simulink model "master_thesis_simulink"  (R2022a)
settings: Solver=VariableStepAuto  StartTime=0.0  StopTime=p_0p.time(end)  FixedStep=0.001  RelTol=1e-3
values from neighbouring files (symbols this model uses):
  markers_forearm = [0.00210510253906 -0.143263397217 -0.00798474121094]    [markers_forearm.mat]
  markers_shoulder = [0.010127746582 -0.151647644043 -0.0119686279297]    [markers_shoulder.mat]
undefined symbols (not defined in the file or in its folder): arm, DiscIntNeverNeededParam, Discrete, ekf, kf, LS, m, markers_hand, n, noise, q0, q0_LS, q0_model, sample_Time, selected, state_observer, Time, tSh_0_0Conf, X, Y, Z
libraries: sm_lib x2029, nesl_utility x1553, robotlib x75, ctrlSharedLib x8
(part 7 of 70)

== system master_thesis_simulink/Experiments/S2_F0_H2/Experiments/KF ==
  p_0' : Inport
  v_0' : Inport  Port=2
  Action Port : ActionPort
  Discrete State-Space : DiscreteStateSpace  Commented=on  A=kf.F  B=kf.G  C=kf.H  D=kf.J  InitialCondition=q0_model - kf.q_eq  SampleTime=sample_Time
  Kalman Filter : MATLAB Function  Commented=on  TreatAsAtomicUnit=on
  Kalman Filter1 : ctrlSharedLib/Kalman Filter  TimeDomain=Discrete-Time  UseCurrentEstimator=on  ModelSource=Individual A, B, C, D matrices  ModelSourceVariable=ss(0.95,1,1,0,1)  A=kf.F  B=kf.G  C=kf.H  D=kf.J  NumberOfStates=1  NumberOfInputs=1  NumberOfOutputs=1  InitialEstimateSource=Dialog  X0=kf.Delta_q0  P0=kf.P0  UseK=off  UseGH=off  NumberOfProcessNoiseInputs=1  G=1  TimeInvariantG=on  H=0  TimeInvariantH=on  Q=noise.Q  TimeInvariantQ=on  R=noise.R  TimeInvariantR=on  N=0  TimeInvariantN=on  AddInputPort=on  AddEnablePort=off  OutputEstimatedY=off  OutputP=off  Ts=sample_Time
  MATLAB Function : MATLAB Function  Commented=on  TreatAsAtomicUnit=on
  R : RandomNumber  Commented=on  Variance=diag(noise.R)  Seed=noise.R_seed  SampleTime=sample_Time
  Scope : Scope  NumInputPorts=2
  Sum1 : Sum  Commented=on  Inputs=++|
  Sum2 : Sum  Commented=on  Inputs=++|
  Sum3 : Sum  Inputs=|+-
  Sum4 : Sum  Inputs=++|
  Sum5 : Sum  Commented=on  Inputs=|++
  Sum6 : Sum  Inputs=|+-
  Terminator1 : Terminator  Commented=on
  Terminator2 : Terminator
  Terminator3 : Terminator
  To Workspace1 : ToWorkspace  VariableName=qk_kf  SaveFormat=Structure With Time  SampleTime=-1
  p_eq : Constant  Value=kf.p_eq  SampleTime=sample_Time
  q_eq : Constant  Commented=on  Value=kf.q_eq  SampleTime=sample_Time
  q_eq1 : Constant  Value=kf.q_eq  SampleTime=sample_Time
  trial : Subsystem  Commented=on
  u_eq : Constant  Value=kf.u_eq  SampleTime=sample_Time
  q_KF : Outport
  wires:
  v_0'/1 -> Sum3/1
  u_eq/1 -> Sum3/2  "u_eqk"
  Sum3/1 -> Kalman Filter1/1, Kalman Filter/2(Delta_uk), trial/1(Delta uk), Sum5/2  "Delta _uk"
  Discrete State-Space/1 -> Sum1/2
  R/1 -> Sum1/1
  Kalman Filter/1(Delta_qk) -> Sum2/2  "Delta qk"
  q_eq/1 -> Sum2/1
  Kalman Filter/2(Pk) -> Terminator1/1
  Sum2/1 -> Scope/1  "kf"
  trial/1(q_OBS) -> Terminator2/1
  trial/2(q_KF) -> Terminator3/1
  Kalman Filter1/1 -> Sum4/2
  q_eq1/1 -> Sum4/1
  Sum4/1 -> q_KF/1, To Workspace1/1, Scope/2  "kf simulink"
  MATLAB Function/1(n_k) -> Sum5/1
  p_0'/1 -> Sum6/1
  p_eq/1 -> Sum6/2  "u_eqk"
  Sum6/1 -> Kalman Filter/1(Delta_pk), Kalman Filter1/2  "Delta_uk"

== system master_thesis_simulink/Experiments/S2_F0_H2/Experiments/LS ==
  p_0' : Inport
  v_0' : Inport  Port=2
  markers shoulder : Inport  Port=3
  markers forearm : Inport  Port=4
  markers hand : Inport  Port=5
  Action Port : ActionPort
  Discrete-Time Integrator : DiscreteIntegrator  InitialCondition=q0_LS  SampleTime=-1  LimitOutput=on  UpperSaturationLimit=4*pi  LowerSaturationLimit=-4*pi  ICPrevOutput=DiscIntNeverNeededParam  ICPrevScaledInput=DiscIntNeverNeededParam
  Gain : Gain  Gain=180/pi
  LS : MATLAB Function  TreatAsAtomicUnit=on
  Scope1 : Scope
  Scope2 : Scope
  error_FK__LS : ToWorkspace  VariableName=error_FK__LS  SaveFormat=Structure With Time  SampleTime=-1
  p_0 - Phi(q_LS) : MATLAB Function  TreatAsAtomicUnit=on
  q_LS : ToWorkspace  VariableName=q_LS  SaveFormat=Structure With Time  SampleTime=-1
  tag scope: q_LS=global
  wires:
  p_0'/1 -> p_0 - Phi(q_LS)/1(p_0)
  p_0 - Phi(q_LS)/1(error_FK) -> error_FK__LS/1, Scope1/1
  Gain/1 -> Scope2/1, q_LS/1  "q_LS [deg]"
  Discrete-Time Integrator/1 -> [q_LS], Gain/1  "q_LS"
  markers hand/1 -> LS/5(hand_variables), p_0 - Phi(q_LS)/5(hand_variables)
  markers forearm/1 -> LS/4(forearm_variables), p_0 - Phi(q_LS)/4(forearm_variables)
  markers shoulder/1 -> LS/3(shoulder_variables), p_0 - Phi(q_LS)/3(shoulder_variables)
  LS/1(qdot_LS) -> Discrete-Time Integrator/1
  [q_LS] -> LS/1(q), p_0 - Phi(q_LS)/2(q_LS)
  v_0'/1 -> LS/2(v_0)

== system master_thesis_simulink/Experiments/S2_F0_H2/Model validation/Display ==
  p_0' : Inport
  p_FK : Inport  Port=2
  Demux : Demux
  Demux1 : Demux
  Mux{,1..3} (4 alike) : Mux  Inputs=2
  Mux8 : Mux
  Scope{,1..3} (4 alike) : Scope
  To Workspace : ToWorkspace  VariableName=p0p_vs_pFK  SaveFormat=Structure With Time  SampleTime=-1
  wires:
  Mux8/1 -> To Workspace/1
  Mux3/1 -> Mux8/4, Scope3/1
  Mux1/1 -> Scope2/1, Mux8/2
  Demux1/4 -> Mux3/2  "M4_FK"
  Demux/4 -> Mux3/1  "M4_0"
  Mux2/1 -> Scope1/1, Mux8/3
  Demux1/3 -> Mux2/2  "M3_FK"
  Demux/3 -> Mux2/1  "M3_0"
  Demux1/2 -> Mux1/2  "M2_FK"
  Demux/2 -> Mux1/1  "M2_0"
  Mux/1 -> Scope/1, Mux8/1
  Demux1/1 -> Mux/2  "M1_FK"
  Demux/1 -> Mux/1  "M1_0"
  p_FK/1 -> Demux1/1
  p_0'/1 -> Demux/1

== system master_thesis_simulink/Experiments/S2_F0_H2/Model validation/Human arm ==
  note: WRIST-HAND
  note: SHOULDER
  note: ELBOW-FOREARM
  note: B_shoulder
  Elbow_joint : Subsystem
  Markers : Subsystem  Commented=on
  Mechanism Configuration : sm_lib/Utilities/Mechanism Configuration  UniformGravity=Constant  GravityVector=[0 0 -9.80665]  GravityUnits=m/s^2  LinearizationDelta=0.001  JointModeTransitionNonlinearIterations=2
  Mux : Mux  Inputs=m
  Mux1 : Mux  Inputs=m
  RightForeArm : Subsystem
  RightHand : Subsystem
  RightShoulder : Subsystem
  RightShoulder_joint : Subsystem
  Solver Configuration1 : nesl_utility/Solver Configuration  PhysicalDomain=network_engine_domain  SubClassName=solver  LeftPortType=input  RightPortType=generic  Tones=[]  Harmonics=[]  SimulateNoise=off  Profile=off  UseLocalSampling=off  EnableSwitchedLinearOptims=on  FrequencyDomain=off  UseCCode=off  RelTol=0.001  AbsTol=0.001  MinStep=1e-09  ToWorkspace=off  RevertToSquareIcSolve=off  NumHomotopyIterations=100  PhasorMode=off  PhasorModeNumHarmonics=1  IndexReductionMethod=DerivativeReplacement  DoDC=off  ResidualTolerance=1e-09  UseLocalSolver=on  LocalSolverChoice=NE_BACKWARD_EULER_ADVANCER  LocalSolverSampleTime=sample_Time  DoFixedCost=on  MaxNonlinIter=3  MaxModeIter=2  ComputeImpulses=off  ImpulseIterations=2  LinearAlgebra=auto  LinearAlgebraNumThread=0  EquationFormulation=NE_TIME_EF  DelaysMemoryBudget=1024  AutomaticFiltering=on  FilteringTimeConstant=0.001  PartitionStorageMethod=AS_NEEDED  PartitionMemoryBudget=1024  PartitionMethod=ROBUST
      settings: SourceProductBaseCode=SS,PW,VE
  World Frame : sm_lib/Frames and Transforms/World Frame
  Wrist_joint : Subsystem
  p : Outport
  pdot : Outport  Port=2
  wires:
  [pdot_4] -> Mux1/4
  [p_4] -> Mux/4
  [pdot_3] -> Mux1/3
  [p_3] -> Mux/3
  [pdot_2] -> Mux1/2
  [p_2] -> Mux/2
  [pdot_1] -> Mux1/1
  [p_1] -> Mux/1
  Mux1/1 -> pdot/1
  Mux/1 -> p/1
  connections:
  RightShoulder_joint/RConn1 -- RightShoulder/LConn1
  RightShoulder/RConn1 -- Elbow_joint/LConn1
  Wrist_joint/LConn1 -- RightForeArm/RConn1
  RightHand/LConn1 -- Wrist_joint/RConn1
  Elbow_joint/RConn1 -- RightForeArm/LConn1
  Solver Configuration1/RConn1 -- RightShoulder_joint/LConn1 -- World Frame/RConn1 -- Mechanism Configuration/RConn1 -- RightShoulder/LConn2 -- RightHand/LConn2 -- RightForeArm/LConn2

== system master_thesis_simulink/Ros2Matlab/S0_F1_H2/Position_M0 & velocity_M0 computation/  ==
  p_W : Inport
  v_W : Inport  Port=2
  quat_02W : Inport  Port=3
  Action Port : ActionPort  ActionPortLabel=if(u1 > 0)
  Mi_M0_POS : MATLAB Function  TreatAsAtomicUnit=on
  p_0' : Outport
  v_0' : Outport  Port=2
  wires:
  v_W/1 -> Mi_M0_POS/2(v_W)
  quat_02W/1 -> Mi_M0_POS/3(quat_02W)
  p_W/1 -> Mi_M0_POS/1(p_W)
  Mi_M0_POS/2(v_0p) -> v_0'/1
  Mi_M0_POS/1(p_0p) -> p_0'/1

== system master_thesis_simulink/Ros2Matlab/S0_F1_H2/Subscriber/M0 ==
  Odom : Subsystem
  Pose : Subsystem
  p0_W : Outport
  v0_W : Outport  Port=2
  quat_02W : Outport  Port=3
  Rp0_W : Outport  Port=4
  Rv0_W : Outport  Port=5
  wires:
  Pose/2(p0_W) -> p0_W/1
  Pose/1(quat_02W) -> quat_02W/1
  Odom/1(v0_W) -> v0_W/1
  Odom/2(Rp0_W) -> Rp0_W/1
  Odom/3(Rv0_W) -> Rv0_W/1

== system master_thesis_simulink/Ros2Matlab/S0_F1_H2/Subscriber/M2 ==
  Odom : Subsystem
  Pose : Subsystem
  p2_W : Outport
  v2_W : Outport  Port=2
  Rp2_W : Outport  Port=3
  Rv2_W : Outport  Port=4
  wires:
  Pose/1(p2_W) -> p2_W/1
  Odom/1(v2_W) -> v2_W/1
  Odom/2(Rp2_W) -> Rp2_W/1
  Odom/3(Rv2_W) -> Rv2_W/1

== system master_thesis_simulink/Ros2Matlab/S0_F1_H2/Subscriber/M3 ==
  Odom : Subsystem
  Pose : Subsystem
  p3_W : Outport
  v3_W : Outport  Port=2
  Rp3_W : Outport  Port=3
  Rv3_W : Outport  Port=4
  wires:
  Odom/1(v3_W) -> v3_W/1
  Pose/1(p3_W) -> p3_W/1
  Odom/2(Rp3_W) -> Rp3_W/1
  Odom/3(Rv3_W) -> Rv3_W/1

== system master_thesis_simulink/Ros2Matlab/S0_F1_H2/Subscriber/M4 ==
  Odom : Subsystem
  Pose : Subsystem
  p4_W : Outport
  v4_W : Outport  Port=2
  Rp4_W : Outport  Port=3
  Rv4_W : Outport  Port=4
  wires:
  Pose/1(p4_W) -> p4_W/1
  Odom/1(v4_W) -> v4_W/1
  Odom/2(Rp4_W) -> Rp4_W/1
  Odom/3(Rv4_W) -> Rv4_W/1

== system master_thesis_simulink/Ros2Matlab/S0_F1_H2/Subscriber/Shoulder_RF ==
  Pose : Subsystem
  pSh_W : Outport
  quat_Sh2W : Outport  Port=2
  wires:
  Pose/2(pSh_W) -> pSh_W/1
  Pose/1(quat_Sh2W) -> quat_Sh2W/1

== system master_thesis_simulink/Ros2Matlab/S0_F1_H2/tSh_0 computation/If Action Subsystem1 ==
  p0_W : Inport
  pSh_W : Inport  Port=2
  quat_02W : Inport  Port=3
  Action Port : ActionPort  ActionPortLabel=if(u1 > 0)
  Mi_M0_POS1 : MATLAB Function  TreatAsAtomicUnit=on
  Scope : Scope
  tSh_0 : Outport
  wires:
  p0_W/1 -> Mi_M0_POS1/1(p0_W)
  quat_02W/1 -> Mi_M0_POS1/3(quat_02W)
  Mi_M0_POS1/1(tSh_0) -> Scope/1, tSh_0/1
  pSh_W/1 -> Mi_M0_POS1/2(pSh_W)

== system master_thesis_simulink/Ros2Matlab/S0_F2_H2/Position_M0 & velocity_M0 computation/  ==
  p_W : Inport
  v_W : Inport  Port=2
  quat_02W : Inport  Port=3
  Action Port : ActionPort  ActionPortLabel=if(u1 > 0)
  Mi_M0_POS : MATLAB Function  TreatAsAtomicUnit=on
  p_0' : Outport
  v_0' : Outport  Port=2
  wires:
  v_W/1 -> Mi_M0_POS/2(v_W)
  quat_02W/1 -> Mi_M0_POS/3(quat_02W)
  p_W/1 -> Mi_M0_POS/1(p_W)
  Mi_M0_POS/2(v_0p) -> v_0'/1
  Mi_M0_POS/1(p_0p) -> p_0'/1

== system master_thesis_simulink/Ros2Matlab/S0_F2_H2/Subscriber/M0 ==
  Odom : Subsystem
  Pose : Subsystem
  p0_W : Outport
  v0_W : Outport  Port=2
  quat_02W : Outport  Port=3
  Rp0_W : Outport  Port=4
  Rv0_W : Outport  Port=5
  wires:
  Pose/2(p0_W) -> p0_W/1
  Pose/1(quat_02W) -> quat_02W/1
  Odom/1(v0_W) -> v0_W/1
  Odom/2(Rp0_W) -> Rp0_W/1
  Odom/3(Rv0_W) -> Rv0_W/1

== system master_thesis_simulink/Ros2Matlab/S0_F2_H2/Subscriber/M1 ==
  Odom : Subsystem
  Pose : Subsystem
  p1_W : Outport
  v1_W : Outport  Port=2
  Rp1_W : Outport  Port=3
  Rv1_W : Outport  Port=4
  wires:
  Odom/1(v1_W) -> v1_W/1
  Pose/1(p1_W) -> p1_W/1
  Odom/2(Rp1_W) -> Rp1_W/1
  Odom/3(Rv1_W) -> Rv1_W/1

== system master_thesis_simulink/Ros2Matlab/S0_F2_H2/Subscriber/M2 ==
  Odom : Subsystem
  Pose : Subsystem
  p2_W : Outport
  v2_W : Outport  Port=2
  Rp2_W : Outport  Port=3
  Rv2_W : Outport  Port=4
  wires:
  Pose/1(p2_W) -> p2_W/1
  Odom/1(v2_W) -> v2_W/1
  Odom/2(Rp2_W) -> Rp2_W/1
  Odom/3(Rv2_W) -> Rv2_W/1

== system master_thesis_simulink/Ros2Matlab/S0_F2_H2/Subscriber/M3 ==
  Odom : Subsystem
  Pose : Subsystem
  p3_W : Outport
  v3_W : Outport  Port=2
  Rp3_W : Outport  Port=3
  Rv3_W : Outport  Port=4
  wires:
  Odom/1(v3_W) -> v3_W/1
  Pose/1(p3_W) -> p3_W/1
  Odom/2(Rp3_W) -> Rp3_W/1
  Odom/3(Rv3_W) -> Rv3_W/1

== system master_thesis_simulink/Ros2Matlab/S0_F2_H2/Subscriber/M4 ==
  Odom : Subsystem
  Pose : Subsystem
  p4_W : Outport
  v4_W : Outport  Port=2
  Rp4_W : Outport  Port=3
  Rv4_W : Outport  Port=4
  wires:
  Pose/1(p4_W) -> p4_W/1
  Odom/1(v4_W) -> v4_W/1
  Odom/2(Rp4_W) -> Rp4_W/1
  Odom/3(Rv4_W) -> Rv4_W/1

== system master_thesis_simulink/Ros2Matlab/S0_F2_H2/Subscriber/Shoulder_RF ==
  Pose : Subsystem
  pSh_W : Outport
  quat_Sh2W : Outport  Port=2
  wires:
  Pose/2(pSh_W) -> pSh_W/1
  Pose/1(quat_Sh2W) -> quat_Sh2W/1

== system master_thesis_simulink/Ros2Matlab/S0_F2_H2/tSh_0 computation/If Action Subsystem1 ==
  p0_W : Inport
  pSh_W : Inport  Port=2
  quat_02W : Inport  Port=3
  Action Port : ActionPort  ActionPortLabel=if(u1 > 0)
  Mi_M0_POS1 : MATLAB Function  TreatAsAtomicUnit=on
  Scope : Scope
  tSh_0 : Outport
  wires:
  p0_W/1 -> Mi_M0_POS1/1(p0_W)
  quat_02W/1 -> Mi_M0_POS1/3(quat_02W)
  Mi_M0_POS1/1(tSh_0) -> Scope/1, tSh_0/1
  pSh_W/1 -> Mi_M0_POS1/2(pSh_W)

== system master_thesis_simulink/Ros2Matlab/S1_F0_H2/Position_M0 & velocity_M0 computation/  ==
  p_W : Inport
  v_W : Inport  Port=2
  quat_02W : Inport  Port=3
  Action Port : ActionPort  ActionPortLabel=if(u1 > 0)
  Mi_M0_POS : MATLAB Function  TreatAsAtomicUnit=on
  p_0' : Outport
  v_0' : Outport  Port=2
  wires:
  v_W/1 -> Mi_M0_POS/2(v_W)
  quat_02W/1 -> Mi_M0_POS/3(quat_02W)
  p_W/1 -> Mi_M0_POS/1(p_W)
  Mi_M0_POS/2(v_0p) -> v_0'/1
  Mi_M0_POS/1(p_0p) -> p_0'/1

== system master_thesis_simulink/Ros2Matlab/S1_F0_H2/Subscriber/M0 ==
  Odom : Subsystem
  Pose : Subsystem
  p0_W : Outport
  v0_W : Outport  Port=2
  quat_02W : Outport  Port=3
  Rp0_W : Outport  Port=4
  Rv0_W : Outport  Port=5
  wires:
  Pose/2(p0_W) -> p0_W/1
  Pose/1(quat_02W) -> quat_02W/1
  Odom/1(v0_W) -> v0_W/1
  Odom/2(Rp0_W) -> Rp0_W/1
  Odom/3(Rv0_W) -> Rv0_W/1

== system master_thesis_simulink/Ros2Matlab/S1_F0_H2/Subscriber/M1 ==
  Odom : Subsystem
  Pose : Subsystem
  p1_W : Outport
  v1_W : Outport  Port=2
  Rp1_W : Outport  Port=3
  Rv1_W : Outport  Port=4
  wires:
  Odom/1(v1_W) -> v1_W/1
  Pose/1(p1_W) -> p1_W/1
  Odom/2(Rp1_W) -> Rp1_W/1
  Odom/3(Rv1_W) -> Rv1_W/1

== system master_thesis_simulink/Ros2Matlab/S1_F0_H2/Subscriber/M3 ==
  Odom : Subsystem
  Pose : Subsystem
  p3_W : Outport
  v3_W : Outport  Port=2
  Rp3_W : Outport  Port=3
  Rv3_W : Outport  Port=4
  wires:
  Odom/1(v3_W) -> v3_W/1
  Pose/1(p3_W) -> p3_W/1
  Odom/2(Rp3_W) -> Rp3_W/1
  Odom/3(Rv3_W) -> Rv3_W/1

== system master_thesis_simulink/Ros2Matlab/S1_F0_H2/Subscriber/M4 ==
  Odom : Subsystem
  Pose : Subsystem
  p4_W : Outport
  v4_W : Outport  Port=2
  Rp4_W : Outport  Port=3
  Rv4_W : Outport  Port=4
  wires:
  Pose/1(p4_W) -> p4_W/1
  Odom/1(v4_W) -> v4_W/1
  Odom/2(Rp4_W) -> Rp4_W/1
  Odom/3(Rv4_W) -> Rv4_W/1

== system master_thesis_simulink/Ros2Matlab/S1_F0_H2/Subscriber/Shoulder_RF ==
  Pose : Subsystem
  pSh_W : Outport
  quat_Sh2W : Outport  Port=2
  wires:
  Pose/2(pSh_W) -> pSh_W/1
  Pose/1(quat_Sh2W) -> quat_Sh2W/1

== system master_thesis_simulink/Ros2Matlab/S1_F0_H2/tSh_0 computation/If Action Subsystem1 ==
  p0_W : Inport
  pSh_W : Inport  Port=2
  quat_02W : Inport  Port=3
  Action Port : ActionPort  ActionPortLabel=if(u1 > 0)
  Mi_M0_POS1 : MATLAB Function  TreatAsAtomicUnit=on
  Scope : Scope
  tSh_0 : Outport
  wires:
  p0_W/1 -> Mi_M0_POS1/1(p0_W)
  quat_02W/1 -> Mi_M0_POS1/3(quat_02W)
  Mi_M0_POS1/1(tSh_0) -> Scope/1, tSh_0/1
  pSh_W/1 -> Mi_M0_POS1/2(pSh_W)

== system master_thesis_simulink/Ros2Matlab/S1_F0_H3/Position_M0 & velocity_M0 computation/  ==
  p_W : Inport
  v_W : Inport  Port=2
  quat_02W : Inport  Port=3
  Action Port : ActionPort  ActionPortLabel=if(u1 > 0)
  Mi_M0_POS : MATLAB Function  TreatAsAtomicUnit=on
  p_0' : Outport
  v_0' : Outport  Port=2
  wires:
  v_W/1 -> Mi_M0_POS/2(v_W)
  quat_02W/1 -> Mi_M0_POS/3(quat_02W)
  p_W/1 -> Mi_M0_POS/1(p_W)
  Mi_M0_POS/2(v_0p) -> v_0'/1
  Mi_M0_POS/1(p_0p) -> p_0'/1

== system master_thesis_simulink/Ros2Matlab/S1_F0_H3/Subscriber/M0 ==
  Odom : Subsystem
  Pose : Subsystem
  p0_W : Outport
  v0_W : Outport  Port=2
  quat_02W : Outport  Port=3
  Rp0_W : Outport  Port=4
  Rv0_W : Outport  Port=5
  wires:
  Pose/2(p0_W) -> p0_W/1
  Pose/1(quat_02W) -> quat_02W/1
  Odom/1(v0_W) -> v0_W/1
  Odom/2(Rp0_W) -> Rp0_W/1
  Odom/3(Rv0_W) -> Rv0_W/1

== system master_thesis_simulink/Ros2Matlab/S1_F0_H3/Subscriber/M1 ==
  Odom : Subsystem
  Pose : Subsystem
  p1_W : Outport
  v1_W : Outport  Port=2
  Rp1_W : Outport  Port=3
  Rv1_W : Outport  Port=4
  wires:
  Odom/1(v1_W) -> v1_W/1
  Pose/1(p1_W) -> p1_W/1
  Odom/2(Rp1_W) -> Rp1_W/1
  Odom/3(Rv1_W) -> Rv1_W/1

== system master_thesis_simulink/Ros2Matlab/S1_F0_H3/Subscriber/M2 ==
  Odom : Subsystem
  Pose : Subsystem
  p2_W : Outport
  v2_W : Outport  Port=2
  Rp2_W : Outport  Port=3
  Rv2_W : Outport  Port=4
  wires:
  Pose/1(p2_W) -> p2_W/1
  Odom/1(v2_W) -> v2_W/1
  Odom/2(Rp2_W) -> Rp2_W/1
  Odom/3(Rv2_W) -> Rv2_W/1

== system master_thesis_simulink/Ros2Matlab/S1_F0_H3/Subscriber/M3 ==
  Odom : Subsystem
  Pose : Subsystem
  p3_W : Outport
  v3_W : Outport  Port=2
  Rp3_W : Outport  Port=3
  Rv3_W : Outport  Port=4
  wires:
  Odom/1(v3_W) -> v3_W/1
  Pose/1(p3_W) -> p3_W/1
  Odom/2(Rp3_W) -> Rp3_W/1
  Odom/3(Rv3_W) -> Rv3_W/1

== system master_thesis_simulink/Ros2Matlab/S1_F0_H3/Subscriber/M4 ==
  Odom : Subsystem
  Pose : Subsystem
  p4_W : Outport
  v4_W : Outport  Port=2
  Rp4_W : Outport  Port=3
  Rv4_W : Outport  Port=4
  wires:
  Pose/1(p4_W) -> p4_W/1
  Odom/1(v4_W) -> v4_W/1
  Odom/2(Rp4_W) -> Rp4_W/1
  Odom/3(Rv4_W) -> Rv4_W/1

== system master_thesis_simulink/Ros2Matlab/S1_F0_H3/Subscriber/Shoulder_RF ==
  Pose : Subsystem
  pSh_W : Outport
  quat_Sh2W : Outport  Port=2
  wires:
  Pose/2(pSh_W) -> pSh_W/1
  Pose/1(quat_Sh2W) -> quat_Sh2W/1

== system master_thesis_simulink/Ros2Matlab/S1_F0_H3/tSh_0 computation/If Action Subsystem1 ==
  p0_W : Inport
  pSh_W : Inport  Port=2
  quat_02W : Inport  Port=3
  Action Port : ActionPort  ActionPortLabel=if(u1 > 0)
  Mi_M0_POS1 : MATLAB Function  TreatAsAtomicUnit=on
  Scope : Scope
  tSh_0 : Outport
  wires:
  p0_W/1 -> Mi_M0_POS1/1(p0_W)
  quat_02W/1 -> Mi_M0_POS1/3(quat_02W)
  Mi_M0_POS1/1(tSh_0) -> Scope/1, tSh_0/1
  pSh_W/1 -> Mi_M0_POS1/2(pSh_W)

== system master_thesis_simulink/Ros2Matlab/S1_F1_H2/Position_M0 & velocity_M0 computation/  ==
  p_W : Inport
  v_W : Inport  Port=2
  quat_02W : Inport  Port=3
  Action Port : ActionPort  ActionPortLabel=if(u1 > 0)
  Mi_M0_POS : MATLAB Function  TreatAsAtomicUnit=on
  p_0' : Outport
  v_0' : Outport  Port=2
  wires:
  v_W/1 -> Mi_M0_POS/2(v_W)
  quat_02W/1 -> Mi_M0_POS/3(quat_02W)
  p_W/1 -> Mi_M0_POS/1(p_W)
  Mi_M0_POS/2(v_0p) -> v_0'/1
  Mi_M0_POS/1(p_0p) -> p_0'/1

== system master_thesis_simulink/Ros2Matlab/S1_F1_H2/Subscriber/M0 ==
  Odom : Subsystem
  Pose : Subsystem
  p0_W : Outport
  v0_W : Outport  Port=2
  quat_02W : Outport  Port=3
  Rp0_W : Outport  Port=4
  Rv0_W : Outport  Port=5
  wires:
  Pose/2(p0_W) -> p0_W/1
  Pose/1(quat_02W) -> quat_02W/1
  Odom/1(v0_W) -> v0_W/1
  Odom/2(Rp0_W) -> Rp0_W/1
  Odom/3(Rv0_W) -> Rv0_W/1

== system master_thesis_simulink/Ros2Matlab/S1_F1_H2/Subscriber/M1 ==
  Odom : Subsystem
  Pose : Subsystem
  p1_W : Outport
  v1_W : Outport  Port=2
  Rp1_W : Outport  Port=3
  Rv1_W : Outport  Port=4
  wires:
  Odom/1(v1_W) -> v1_W/1
  Pose/1(p1_W) -> p1_W/1
  Odom/2(Rp1_W) -> Rp1_W/1
  Odom/3(Rv1_W) -> Rv1_W/1

== system master_thesis_simulink/Ros2Matlab/S1_F1_H2/Subscriber/M2 ==
  Odom : Subsystem
  Pose : Subsystem
  p2_W : Outport
  v2_W : Outport  Port=2
  Rp2_W : Outport  Port=3
  Rv2_W : Outport  Port=4
  wires:
  Pose/1(p2_W) -> p2_W/1
  Odom/1(v2_W) -> v2_W/1
  Odom/2(Rp2_W) -> Rp2_W/1
  Odom/3(Rv2_W) -> Rv2_W/1

== system master_thesis_simulink/Ros2Matlab/S1_F1_H2/Subscriber/M3 ==
  Odom : Subsystem
  Pose : Subsystem
  p3_W : Outport
  v3_W : Outport  Port=2
  Rp3_W : Outport  Port=3
  Rv3_W : Outport  Port=4
  wires:
  Odom/1(v3_W) -> v3_W/1
  Pose/1(p3_W) -> p3_W/1
  Odom/2(Rp3_W) -> Rp3_W/1
  Odom/3(Rv3_W) -> Rv3_W/1

== system master_thesis_simulink/Ros2Matlab/S1_F1_H2/Subscriber/M4 ==
  Odom : Subsystem
  Pose : Subsystem
  p4_W : Outport
  v4_W : Outport  Port=2
  Rp4_W : Outport  Port=3
  Rv4_W : Outport  Port=4
  wires:
  Pose/1(p4_W) -> p4_W/1
  Odom/1(v4_W) -> v4_W/1
  Odom/2(Rp4_W) -> Rp4_W/1
  Odom/3(Rv4_W) -> Rv4_W/1

== system master_thesis_simulink/Ros2Matlab/S1_F1_H2/Subscriber/Shoulder_RF ==
  Pose : Subsystem
  pSh_W : Outport
  quat_Sh2W : Outport  Port=2
  wires:
  Pose/2(pSh_W) -> pSh_W/1
  Pose/1(quat_Sh2W) -> quat_Sh2W/1

== system master_thesis_simulink/Ros2Matlab/S1_F1_H2/tSh_0 computation/If Action Subsystem1 ==
  p0_W : Inport
  pSh_W : Inport  Port=2
  quat_02W : Inport  Port=3
  Action Port : ActionPort  ActionPortLabel=if(u1 > 0)
  Mi_M0_POS1 : MATLAB Function  TreatAsAtomicUnit=on
  Scope : Scope
  tSh_0 : Outport
  wires:
  p0_W/1 -> Mi_M0_POS1/1(p0_W)
  quat_02W/1 -> Mi_M0_POS1/3(quat_02W)
  Mi_M0_POS1/1(tSh_0) -> Scope/1, tSh_0/1
  pSh_W/1 -> Mi_M0_POS1/2(pSh_W)

== system master_thesis_simulink/Ros2Matlab/S1_F2_H2/Position_M0 & velocity_M0 computation/  ==
  p_W : Inport
  v_W : Inport  Port=2
  quat_02W : Inport  Port=3
  Action Port : ActionPort  ActionPortLabel=if(u1 > 0)
  Mi_M0_POS : MATLAB Function  TreatAsAtomicUnit=on
  p_0' : Outport
  v_0' : Outport  Port=2
  wires:
  Mi_M0_POS/1(p_0p) -> p_0'/1
  Mi_M0_POS/2(v_0p) -> v_0'/1
  p_W/1 -> Mi_M0_POS/1(p_W)
  quat_02W/1 -> Mi_M0_POS/3(quat_02W)
  v_W/1 -> Mi_M0_POS/2(v_W)

== system master_thesis_simulink/Ros2Matlab/S1_F2_H2/Subscriber/M0 ==
  Odom : Subsystem
  Pose : Subsystem
  p0_W : Outport
  v0_W : Outport  Port=2
  quat_02W : Outport  Port=3
  Rp0_W : Outport  Port=4
  Rv0_W : Outport  Port=5
  wires:
  Odom/3(Rv0_W) -> Rv0_W/1
  Odom/2(Rp0_W) -> Rp0_W/1
  Odom/1(v0_W) -> v0_W/1
  Pose/1(quat_02W) -> quat_02W/1
  Pose/2(p0_W) -> p0_W/1

== system master_thesis_simulink/Ros2Matlab/S1_F2_H2/Subscriber/M1 ==
  Odom : Subsystem
  Pose : Subsystem
  p1_W : Outport
  v1_W : Outport  Port=2
  Rp1_W : Outport  Port=3
  Rv1_W : Outport  Port=4
  wires:
  Odom/3(Rv1_W) -> Rv1_W/1
  Odom/2(Rp1_W) -> Rp1_W/1
  Pose/1(p1_W) -> p1_W/1
  Odom/1(v1_W) -> v1_W/1

== system master_thesis_simulink/Ros2Matlab/S1_F2_H2/Subscriber/M2 ==
  Odom : Subsystem
  Pose : Subsystem
  p2_W : Outport
  v2_W : Outport  Port=2
  Rp2_W : Outport  Port=3
  Rv2_W : Outport  Port=4
  wires:
  Odom/3(Rv2_W) -> Rv2_W/1
  Odom/2(Rp2_W) -> Rp2_W/1
  Odom/1(v2_W) -> v2_W/1
  Pose/1(p2_W) -> p2_W/1

== system master_thesis_simulink/Ros2Matlab/S1_F2_H2/Subscriber/M3 ==
  Odom : Subsystem
  Pose : Subsystem
  p3_W : Outport
  v3_W : Outport  Port=2
  Rp3_W : Outport  Port=3
  Rv3_W : Outport  Port=4
  wires:
  Odom/3(Rv3_W) -> Rv3_W/1
  Odom/2(Rp3_W) -> Rp3_W/1
  Pose/1(p3_W) -> p3_W/1
  Odom/1(v3_W) -> v3_W/1

== system master_thesis_simulink/Ros2Matlab/S1_F2_H2/Subscriber/M4 ==
  Odom : Subsystem
  Pose : Subsystem
  p4_W : Outport
  v4_W : Outport  Port=2
  Rp4_W : Outport  Port=3
  Rv4_W : Outport  Port=4
  wires:
  Odom/3(Rv4_W) -> Rv4_W/1
  Odom/2(Rp4_W) -> Rp4_W/1
  Odom/1(v4_W) -> v4_W/1
  Pose/1(p4_W) -> p4_W/1

== system master_thesis_simulink/Ros2Matlab/S1_F2_H2/Subscriber/M5 ==
  Odom : Subsystem
  Pose : Subsystem
  p2_W : Outport
  v2_W : Outport  Port=2
  Rp2_W : Outport  Port=3
  Rv2_W : Outport  Port=4
  wires:
  Pose/1(p5_W) -> p2_W/1
  Odom/1(v2_W) -> v2_W/1
  Odom/2(Rp2_W) -> Rp2_W/1
  Odom/3(Rv2_W) -> Rv2_W/1

== system master_thesis_simulink/Ros2Matlab/S1_F2_H2/Subscriber/Shoulder_RF ==
  Pose : Subsystem
  pSh_W : Outport
  quat_Sh2W : Outport  Port=2
  wires:
  Pose/1(quat_Sh2W) -> quat_Sh2W/1
  Pose/2(pSh_W) -> pSh_W/1

== system master_thesis_simulink/Ros2Matlab/S1_F2_H2/tSh_0 computation/If Action Subsystem1 ==
  p0_W : Inport
  pSh_W : Inport  Port=2
  quat_02W : Inport  Port=3
  Action Port : ActionPort  ActionPortLabel=if(u1 > 0)
  Mi_M0_POS1 : MATLAB Function  TreatAsAtomicUnit=on
  Scope : Scope
  tSh_0 : Outport
  wires:
  pSh_W/1 -> Mi_M0_POS1/2(pSh_W)
  Mi_M0_POS1/1(tSh_0) -> tSh_0/1, Scope/1
  quat_02W/1 -> Mi_M0_POS1/3(quat_02W)
  p0_W/1 -> Mi_M0_POS1/1(p0_W)

== system master_thesis_simulink/Ros2Matlab/S2_F0_H2/Position_M0 & velocity_M0 computation/  ==
  p_W : Inport
  v_W : Inport  Port=2
  quat_02W : Inport  Port=3
  Action Port : ActionPort  ActionPortLabel=if(u1 > 0)
  Mi_M0_POS : MATLAB Function  TreatAsAtomicUnit=on
  p_0' : Outport
  v_0' : Outport  Port=2
  wires:
  v_W/1 -> Mi_M0_POS/2(v_W)
  quat_02W/1 -> Mi_M0_POS/3(quat_02W)
  p_W/1 -> Mi_M0_POS/1(p_W)
  Mi_M0_POS/2(v_0p) -> v_0'/1
  Mi_M0_POS/1(p_0p) -> p_0'/1

== system master_thesis_simulink/Ros2Matlab/S2_F0_H2/Subscriber/M0 ==
  Odom : Subsystem
  Pose : Subsystem
  p0_W : Outport
  v0_W : Outport  Port=2
  quat_02W : Outport  Port=3
  Rp0_W : Outport  Port=4
  Rv0_W : Outport  Port=5
  wires:
  Pose/2(p0_W) -> p0_W/1
  Pose/1(quat_02W) -> quat_02W/1
  Odom/1(v0_W) -> v0_W/1
  Odom/2(Rp0_W) -> Rp0_W/1
  Odom/3(Rv0_W) -> Rv0_W/1

== system master_thesis_simulink/Ros2Matlab/S2_F0_H2/Subscriber/M1 ==
  Odom : Subsystem
  Pose : Subsystem
  p1_W : Outport
  v1_W : Outport  Port=2
  Rp1_W : Outport  Port=3
  Rv1_W : Outport  Port=4
  wires:
  Odom/1(v1_W) -> v1_W/1
  Pose/1(p1_W) -> p1_W/1
  Odom/2(Rp1_W) -> Rp1_W/1
  Odom/3(Rv1_W) -> Rv1_W/1

== system master_thesis_simulink/Ros2Matlab/S2_F0_H2/Subscriber/M2 ==
  Odom : Subsystem
  Pose : Subsystem
  p2_W : Outport
  v2_W : Outport  Port=2
  Rp2_W : Outport  Port=3
  Rv2_W : Outport  Port=4
  wires:
  Pose/1(p2_W) -> p2_W/1
  Odom/1(v2_W) -> v2_W/1
  Odom/2(Rp2_W) -> Rp2_W/1
  Odom/3(Rv2_W) -> Rv2_W/1

== system master_thesis_simulink/Ros2Matlab/S2_F0_H2/Subscriber/M3 ==
  Odom : Subsystem
  Pose : Subsystem
  p3_W : Outport
  v3_W : Outport  Port=2
  Rp3_W : Outport  Port=3
  Rv3_W : Outport  Port=4
  wires:
  Odom/1(v3_W) -> v3_W/1
  Pose/1(p3_W) -> p3_W/1
  Odom/2(Rp3_W) -> Rp3_W/1
  Odom/3(Rv3_W) -> Rv3_W/1

== system master_thesis_simulink/Ros2Matlab/S2_F0_H2/Subscriber/M4 ==
  Odom : Subsystem
  Pose : Subsystem
  p4_W : Outport
  v4_W : Outport  Port=2
  Rp4_W : Outport  Port=3
  Rv4_W : Outport  Port=4
  wires:
  Pose/1(p4_W) -> p4_W/1
  Odom/1(v4_W) -> v4_W/1
  Odom/2(Rp4_W) -> Rp4_W/1
  Odom/3(Rv4_W) -> Rv4_W/1

== system master_thesis_simulink/Ros2Matlab/S2_F0_H2/Subscriber/Shoulder_RF ==
  Pose : Subsystem
  pSh_W : Outport
  quat_Sh2W : Outport  Port=2
  wires:
  Pose/2(pSh_W) -> pSh_W/1
  Pose/1(quat_Sh2W) -> quat_Sh2W/1

== system master_thesis_simulink/Ros2Matlab/S2_F0_H2/tSh_0 computation/If Action Subsystem1 ==
  p0_W : Inport
  pSh_W : Inport  Port=2
  quat_02W : Inport  Port=3
  Action Port : ActionPort  ActionPortLabel=if(u1 > 0)
  Mi_M0_POS1 : MATLAB Function  TreatAsAtomicUnit=on
  Scope : Scope
  tSh_0 : Outport
  wires:
  p0_W/1 -> Mi_M0_POS1/1(p0_W)
  quat_02W/1 -> Mi_M0_POS1/3(quat_02W)
  Mi_M0_POS1/1(tSh_0) -> Scope/1, tSh_0/1
  pSh_W/1 -> Mi_M0_POS1/2(pSh_W)

== system master_thesis_simulink/System/Human arm/Markers/M1 ==
  Marker 1 : sm_lib/Body Elements/Spherical Solid  GraphicAmbientColor=[0.15 0.15 0.15 1.0]  BasedOnType=Density  CenterOfMass=[0 0 0]  CenterOfMassUnits=m  GraphicDiffuseColor=[1.0 0.2 0.2]  Density=1000  DensityUnits=kg/m^3  DoExposeReferenceFrame=on  GraphicEmissiveColor=[0.0 0.0 0.0 1.0]  ExportEntireGeometry=off  SerializedExposedGeometries=<ExposedGeometries/>  SerializedFrames=<Frames/>  MarkerShape=Sphere  MarkerSize=10  GraphicType=FromGeometry  InertiaType=CalculateFromGeometry  Mass=1  MassUnits=kg  MomentsOfInertia=[1 1 1]  MomentsOfInertiaUnits=kg*m^2  GraphicOpacity=1.0  ProductsOfInertia=[0 0 0]  ProductsOfInertiaUnits=kg*m^2  GraphicShininess=75  GraphicSpecularColor=[0.5 0.5 0.5 1.0]  SphereRadius=arm.markers.radius  SphereRadiusUnits=m  GraphicVisPropType=SimpleVisualProperties
  Mux11 : Mux  Inputs=3
  Mux3 : Mux  Inputs=3
  PS-Simulink Converter{9..11,34..36} (6 alike) : nesl_utility/PS-Simulink Converter  PhysicalDomain=network_engine_domain  SubClassName=ps_output  LeftPortType=input  RightPortType=output  PseudoPeriodic=off  Frequencies=[]  VectorFormat=inherit  Unit=inherit  AffineConversion=off
      settings: SourceProductBaseCode=SS,PW,VE
  Transform Sensor3 : sm_lib/Frames and Transforms/Transform Sensor  MeasurementFrame=World  SenseAngle=off  SenseAxis=off  SenseAngle1=off  SenseAngle2=off  SenseAngle3=off  SenseQ=off  SenseR=off  SenseOmegaX=off  SenseOmegaY=off  SenseOmegaZ=off  SenseOmega1=off  SenseOmega2=off  SenseOmega3=off  SenseQDot=off  SenseRDot=off  SenseAlphaX=off  SenseAlphaY=off  SenseAlphaZ=off  SenseAlpha1=off  SenseAlpha2=off  SenseAlpha3=off  SenseQDDot=off  SenseRDDot=off  SenseX=on  SenseY=on  SenseZ=on  SenseRad=off  SenseAzim=off  SenseDist=off  SenseInc=off  SenseXDot=on  SenseYDot=on  SenseZDot=on  SenseRadDot=off  SenseAzimDot=off  SenseDistDot=off  SenseIncDot=off  SenseXDDot=off  SenseYDDot=off  SenseZDDot=off  SenseRadDDot=off  SenseAzimDDot=off  SenseDistDDot=off  SenseIncDDot=off
  translation_R2Base : sm_lib/Frames and Transforms/Rigid Transform  TranslationMethod=Cartesian  TranslationStandardOffset=0  TranslationLengthUnit=m  TranslationStandardAxis=+Z  TranslationCartesianOffset=[arm.shoulder.radius+arm.markers.radius 0 0]  TranslationROffset=0  TranslationROffsetUnits=m  TranslationZOffset=0  TranslationZOffsetUnits=m  TranslationThetaOffset=0  TranslationThetaOffsetUnits=deg  RotationMethod=None  RotationAngleUnits=rad  RotationStandardAxis=+Z  RotationAngle=pi/2  RotationArbitraryAxis=[1 0 0]  FollAlignAxisA=+X  BaseAlignAxisA=+Y  FollAlignAxisB=+Y  BaseAlignAxisB=+Z  RotationSequenceAxes=BaseAxes  RotationSequence=XYZ  RotationSequenceAngles=[pi/2, 0, 0]  RotationSequenceAnglesUnits=rad  RotationMatrix=[1 0 0; 0 1 0; 0 0 1]
  translation_x : sm_lib/Frames and Transforms/Rigid Transform  TranslationMethod=Cartesian  TranslationStandardOffset=0  TranslationLengthUnit=m  TranslationStandardAxis=+Z  TranslationCartesianOffset=[arm.shoulder.radius+arm.markers.radius 0 0]  TranslationROffset=0  TranslationROffsetUnits=m  TranslationZOffset=0  TranslationZOffsetUnits=m  TranslationThetaOffset=0  TranslationThetaOffsetUnits=deg  RotationMethod=None  RotationAngleUnits=rad  RotationStandardAxis=+Z  RotationAngle=pi/2  RotationArbitraryAxis=[1 0 0]  FollAlignAxisA=+X  BaseAlignAxisA=+Y  FollAlignAxisB=+Y  BaseAlignAxisB=+Z  RotationSequenceAxes=BaseAxes  RotationSequence=XYZ  RotationSequenceAngles=[pi/2, 0, 0]  RotationSequenceAnglesUnits=rad  RotationMatrix=[1 0 0; 0 1 0; 0 0 1]
  translation_y : sm_lib/Frames and Transforms/Rigid Transform  TranslationMethod=Cartesian  TranslationStandardOffset=0  TranslationLengthUnit=m  TranslationStandardAxis=+Z  TranslationCartesianOffset=[0 arm.shoulder.length/4 0]  TranslationROffset=0  TranslationROffsetUnits=m  TranslationZOffset=0  TranslationZOffsetUnits=m  TranslationThetaOffset=0  TranslationThetaOffsetUnits=deg  RotationMethod=None  RotationAngleUnits=rad  RotationStandardAxis=+Z  RotationAngle=pi/2  RotationArbitraryAxis=[1 0 0]  FollAlignAxisA=+X  BaseAlignAxisA=+Y  FollAlignAxisB=+Y  BaseAlignAxisB=+Z  RotationSequenceAxes=BaseAxes  RotationSequence=XYZ  RotationSequenceAngles=[pi/2, 0, 0]  RotationSequenceAnglesUnits=rad  RotationMatrix=[1 0 0; 0 1 0; 0 0 1]
  translation_z : sm_lib/Frames and Transforms/Rigid Transform  TranslationMethod=Cartesian  TranslationStandardOffset=0  TranslationLengthUnit=m  TranslationStandardAxis=+Z  TranslationCartesianOffset=[0 0 0]  TranslationROffset=0  TranslationROffsetUnits=m  TranslationZOffset=0  TranslationZOffsetUnits=m  TranslationThetaOffset=0  TranslationThetaOffsetUnits=deg  RotationMethod=None  RotationAngleUnits=rad  RotationStandardAxis=+Z  RotationAngle=pi/2  RotationArbitraryAxis=[1 0 0]  FollAlignAxisA=+X  BaseAlignAxisA=+Y  FollAlignAxisB=+Y  BaseAlignAxisB=+Z  RotationSequenceAxes=BaseAxes  RotationSequence=XYZ  RotationSequenceAngles=[pi/2, 0, 0]  RotationSequenceAnglesUnits=rad  RotationMatrix=[1 0 0; 0 1 0; 0 0 1]
  W : PMIOPort  Side=Left
  R : PMIOPort  Port=2  Side=Left
  p_1 : Outport
  pdot_1 : Outport  Port=2
  wires:
  Mux11/1 -> pdot_1/1
  PS-Simulink Converter9/1 -> Mux11/1  "M1_velx"
  PS-Simulink Converter35/1 -> Mux3/2  "M1_posy"
  PS-Simulink Converter10/1 -> Mux11/2  "M1_vely"
  Mux3/1 -> p_1/1
  PS-Simulink Converter11/1 -> Mux11/3  "M1_velz"
  PS-Simulink Converter34/1 -> Mux3/1  "M1_posx"
  PS-Simulink Converter36/1 -> Mux3/3  "M1_posz"
  connections:
  PS-Simulink Converter9/LConn1 -- Transform Sensor3/RConn5
  PS-Simulink Converter34/LConn1 -- Transform Sensor3/RConn2
  PS-Simulink Converter11/LConn1 -- Transform Sensor3/RConn7
  PS-Simulink Converter10/LConn1 -- Transform Sensor3/RConn6
  translation_z/LConn1 -- translation_y/RConn1
  W/RConn1 -- Transform Sensor3/LConn1
  PS-Simulink Converter35/LConn1 -- Transform Sensor3/RConn3
  Transform Sensor3/RConn4 -- PS-Simulink Converter36/LConn1
  translation_y/LConn1 -- translation_x/RConn1
  translation_R2Base/LConn1 -- R/RConn1
  translation_R2Base/RConn1 -- translation_x/LConn1
  Marker 1/RConn1 -- Transform Sensor3/RConn1 -- translation_z/RConn1

== system master_thesis_simulink/System/Human arm/RightHand/Markers ==
  M1 : Subsystem
  M2 : Subsystem
  W : PMIOPort  Side=Left
  R : PMIOPort  Port=2  Side=Left
  tag scope: p_2=global, p_3=global, pdot_2=global, pdot_3=global
  wires:
  M1/2(pdot_1) -> [pdot_2]
  M1/1(p_1) -> [p_2]
  M2/1(p_1) -> [p_3]
  M2/2(pdot_1) -> [pdot_3]
  connections:
  M1/LConn1 -- W/RConn1 -- M2/LConn1
  M1/LConn2 -- R/RConn1 -- M2/LConn2

== system master_thesis_simulink/System/Human arm/RightShoulder/Markers ==
  M1 : Subsystem
  W : PMIOPort  Side=Left
  R : PMIOPort  Port=2  Side=Left
  tag scope: p_1=global, pdot_1=global
  wires:
  M1/2(pdot_1) -> [pdot_1]
  M1/1(p_1) -> [p_1]
  connections:
  W/RConn1 -- M1/LConn1
  R/RConn1 -- M1/LConn2

== system master_thesis_simulink/System/Human arm/RightShoulder_joint/Sx_Sy ==
  jRightShoulder_rotx_AxisInvTransform : sm_lib/Frames and Transforms/Rigid Transform  TranslationMethod=Cartesian  TranslationStandardOffset=0  TranslationLengthUnit=m  TranslationStandardAxis=+Z  TranslationCartesianOffset=[0, 0, 0]  TranslationROffset=0  TranslationROffsetUnits=m  TranslationZOffset=0  TranslationZOffsetUnits=m  TranslationThetaOffset=0  TranslationThetaOffsetUnits=deg  RotationMethod=ArbitraryAxis  RotationAngleUnits=rad  RotationStandardAxis=+Z  RotationAngle=pi/2  RotationArbitraryAxis=[0, 1, 0]  FollAlignAxisA=+X  BaseAlignAxisA=+Y  FollAlignAxisB=+Y  BaseAlignAxisB=+Z  RotationSequenceAxes=FollowerAxes  RotationSequence=XYX  RotationSequenceAngles=[0 0 0]  RotationSequenceAnglesUnits=deg  RotationMatrix=[1 0 0; 0 1 0; 0 0 1]
  jRightShoulder_rotx_AxisInvTransform1 : sm_lib/Frames and Transforms/Rigid Transform  TranslationMethod=Cartesian  TranslationStandardOffset=0  TranslationLengthUnit=m  TranslationStandardAxis=+Z  TranslationCartesianOffset=[0, 0, 0]  TranslationROffset=0  TranslationROffsetUnits=m  TranslationZOffset=0  TranslationZOffsetUnits=m  TranslationThetaOffset=0  TranslationThetaOffsetUnits=deg  RotationMethod=ArbitraryAxis  RotationAngleUnits=rad  RotationStandardAxis=+Z  RotationAngle=pi/2  RotationArbitraryAxis=[0, 0, 1]  FollAlignAxisA=+X  BaseAlignAxisA=+Y  FollAlignAxisB=+Y  BaseAlignAxisB=+Z  RotationSequenceAxes=FollowerAxes  RotationSequence=XYX  RotationSequenceAngles=[0 0 0]  RotationSequenceAnglesUnits=deg  RotationMatrix=[1 0 0; 0 1 0; 0 0 1]
  Sx : PMIOPort  Side=Left
  Sy : PMIOPort  Port=2  Side=Right
  connections:
  Sx/RConn1 -- jRightShoulder_rotx_AxisInvTransform/LConn1
  jRightShoulder_rotx_AxisInvTransform/RConn1 -- jRightShoulder_rotx_AxisInvTransform1/LConn1
  jRightShoulder_rotx_AxisInvTransform1/RConn1 -- Sy/RConn1

== system master_thesis_simulink/System/Human arm/RightShoulder_joint/Sy_Sz ==
  jRightShoulder_roty_AxisInvTransform : sm_lib/Frames and Transforms/Rigid Transform  TranslationMethod=Cartesian  TranslationStandardOffset=0  TranslationLengthUnit=m  TranslationStandardAxis=+Z  TranslationCartesianOffset=[0, 0, 0]  TranslationROffset=0  TranslationROffsetUnits=m  TranslationZOffset=0  TranslationZOffsetUnits=m  TranslationThetaOffset=0  TranslationThetaOffsetUnits=deg  RotationMethod=ArbitraryAxis  RotationAngleUnits=rad  RotationStandardAxis=+Z  RotationAngle=pi/2  RotationArbitraryAxis=[0, 1, 0]  FollAlignAxisA=+X  BaseAlignAxisA=+Y  FollAlignAxisB=+Y  BaseAlignAxisB=+Z  RotationSequenceAxes=FollowerAxes  RotationSequence=XYX  RotationSequenceAngles=[0 0 0]  RotationSequenceAnglesUnits=deg  RotationMatrix=[1 0 0; 0 1 0; 0 0 1]
  jRightShoulder_roty_AxisInvTransform1 : sm_lib/Frames and Transforms/Rigid Transform  TranslationMethod=Cartesian  TranslationStandardOffset=0  TranslationLengthUnit=m  TranslationStandardAxis=+Z  TranslationCartesianOffset=[0, 0, 0]  TranslationROffset=0  TranslationROffsetUnits=m  TranslationZOffset=0  TranslationZOffsetUnits=m  TranslationThetaOffset=0  TranslationThetaOffsetUnits=deg  RotationMethod=ArbitraryAxis  RotationAngleUnits=rad  RotationStandardAxis=+Z  RotationAngle=pi/2  RotationArbitraryAxis=[0, 0, 1]  FollAlignAxisA=+X  BaseAlignAxisA=+Y  FollAlignAxisB=+Y  BaseAlignAxisB=+Z  RotationSequenceAxes=FollowerAxes  RotationSequence=XYX  RotationSequenceAngles=[0 0 0]  RotationSequenceAnglesUnits=deg  RotationMatrix=[1 0 0; 0 1 0; 0 0 1]
  Sy : PMIOPort  Side=Left
  Sz : PMIOPort  Port=2  Side=Right
  connections:
  Sy/RConn1 -- jRightShoulder_roty_AxisInvTransform/LConn1
  jRightShoulder_roty_AxisInvTransform/RConn1 -- jRightShoulder_roty_AxisInvTransform1/LConn1
  jRightShoulder_roty_AxisInvTransform1/RConn1 -- Sz/RConn1

== system master_thesis_simulink/System/Human arm/RightShoulder_joint/W_Sx ==
  jRightShoulder_rotx_OriginTransform : sm_lib/Frames and Transforms/Rigid Transform  TranslationMethod=Cartesian  TranslationStandardOffset=0  TranslationLengthUnit=m  TranslationStandardAxis=+Z  TranslationCartesianOffset=[0, 0, 0]  TranslationROffset=0  TranslationROffsetUnits=m  TranslationZOffset=0  TranslationZOffsetUnits=m  TranslationThetaOffset=0  TranslationThetaOffsetUnits=deg  RotationMethod=ArbitraryAxis  RotationAngleUnits=rad  RotationStandardAxis=+Z  RotationAngle=pi/2  RotationArbitraryAxis=[0 0 1]  FollAlignAxisA=+X  BaseAlignAxisA=+Y  FollAlignAxisB=+Y  BaseAlignAxisB=+Z  RotationSequenceAxes=BaseAxes  RotationSequence=XYZ  RotationSequenceAngles=[0, pi/2, 0]  RotationSequenceAnglesUnits=rad  RotationMatrix=[1 0 0; 0 1 0; 0 0 1]
  jRightShoulder_rotx_OriginTransform1 : sm_lib/Frames and Transforms/Rigid Transform  TranslationMethod=Cartesian  TranslationStandardOffset=0  TranslationLengthUnit=m  TranslationStandardAxis=+Z  TranslationCartesianOffset=[0, 0, 0]  TranslationROffset=0  TranslationROffsetUnits=m  TranslationZOffset=0  TranslationZOffsetUnits=m  TranslationThetaOffset=0  TranslationThetaOffsetUnits=deg  RotationMethod=ArbitraryAxis  RotationAngleUnits=rad  RotationStandardAxis=+Z  RotationAngle=pi/2  RotationArbitraryAxis=[1 0 0]  FollAlignAxisA=+X  BaseAlignAxisA=+Y  FollAlignAxisB=+Y  BaseAlignAxisB=+Z  RotationSequenceAxes=BaseAxes  RotationSequence=XYZ  RotationSequenceAngles=[0, pi/2, 0]  RotationSequenceAnglesUnits=rad  RotationMatrix=[1 0 0; 0 1 0; 0 0 1]
  W : PMIOPort  Side=Left
  Sx : PMIOPort  Port=2  Side=Right
  connections:
  W/RConn1 -- jRightShoulder_rotx_OriginTransform/LConn1
  jRightShoulder_rotx_OriginTransform1/LConn1 -- jRightShoulder_rotx_OriginTransform/RConn1
  jRightShoulder_rotx_OriginTransform1/RConn1 -- Sx/RConn1

== system master_thesis_simulink/System/Human arm/Wrist_joint/F_elbow__Wx ==
  jRightShoulder_rotx_OriginTransform : sm_lib/Frames and Transforms/Rigid Transform  TranslationMethod=Cartesian  TranslationStandardOffset=0  TranslationLengthUnit=m  TranslationStandardAxis=+Z  TranslationCartesianOffset=[0, 0, 0]  TranslationROffset=0  TranslationROffsetUnits=m  TranslationZOffset=0  TranslationZOffsetUnits=m  TranslationThetaOffset=0  TranslationThetaOffsetUnits=deg  RotationMethod=ArbitraryAxis  RotationAngleUnits=rad  RotationStandardAxis=+Z  RotationAngle=pi/2  RotationArbitraryAxis=[0 0 1]  FollAlignAxisA=+X  BaseAlignAxisA=+Y  FollAlignAxisB=+Y  BaseAlignAxisB=+Z  RotationSequenceAxes=BaseAxes  RotationSequence=XYZ  RotationSequenceAngles=[0, pi/2, 0]  RotationSequenceAnglesUnits=rad  RotationMatrix=[1 0 0; 0 1 0; 0 0 1]
  jRightShoulder_rotx_OriginTransform1 : sm_lib/Frames and Transforms/Rigid Transform  TranslationMethod=Cartesian  TranslationStandardOffset=0  TranslationLengthUnit=m  TranslationStandardAxis=+Z  TranslationCartesianOffset=[0, 0, 0]  TranslationROffset=0  TranslationROffsetUnits=m  TranslationZOffset=0  TranslationZOffsetUnits=m  TranslationThetaOffset=0  TranslationThetaOffsetUnits=deg  RotationMethod=ArbitraryAxis  RotationAngleUnits=rad  RotationStandardAxis=+Z  RotationAngle=pi/2  RotationArbitraryAxis=[1 0 0]  FollAlignAxisA=+X  BaseAlignAxisA=+Y  FollAlignAxisB=+Y  BaseAlignAxisB=+Z  RotationSequenceAxes=BaseAxes  RotationSequence=XYZ  RotationSequenceAngles=[0, pi/2, 0]  RotationSequenceAnglesUnits=rad  RotationMatrix=[1 0 0; 0 1 0; 0 0 1]
  B_wrist : PMIOPort  Side=Left
  Wx : PMIOPort  Port=2  Side=Right
  connections:
  B_wrist/RConn1 -- jRightShoulder_rotx_OriginTransform/LConn1
  jRightShoulder_rotx_OriginTransform1/LConn1 -- jRightShoulder_rotx_OriginTransform/RConn1
  jRightShoulder_rotx_OriginTransform1/RConn1 -- Wx/RConn1

== system master_thesis_simulink/System/Human arm/Wrist_joint/Wx_Wy ==
  jRightShoulder_rotx_AxisInvTransform2 : sm_lib/Frames and Transforms/Rigid Transform  TranslationMethod=Cartesian  TranslationStandardOffset=0  TranslationLengthUnit=m  TranslationStandardAxis=+Z  TranslationCartesianOffset=[0, 0, 0]  TranslationROffset=0  TranslationROffsetUnits=m  TranslationZOffset=0  TranslationZOffsetUnits=m  TranslationThetaOffset=0  TranslationThetaOffsetUnits=deg  RotationMethod=ArbitraryAxis  RotationAngleUnits=rad  RotationStandardAxis=+Z  RotationAngle=pi/2  RotationArbitraryAxis=[0, 1, 0]  FollAlignAxisA=+X  BaseAlignAxisA=+Y  FollAlignAxisB=+Y  BaseAlignAxisB=+Z  RotationSequenceAxes=FollowerAxes  RotationSequence=XYX  RotationSequenceAngles=[0 0 0]  RotationSequenceAnglesUnits=deg  RotationMatrix=[1 0 0; 0 1 0; 0 0 1]
  jRightShoulder_rotx_AxisInvTransform3 : sm_lib/Frames and Transforms/Rigid Transform  TranslationMethod=Cartesian  TranslationStandardOffset=0  TranslationLengthUnit=m  TranslationStandardAxis=+Z  TranslationCartesianOffset=[0, 0, 0]  TranslationROffset=0  TranslationROffsetUnits=m  TranslationZOffset=0  TranslationZOffsetUnits=m  TranslationThetaOffset=0  TranslationThetaOffsetUnits=deg  RotationMethod=ArbitraryAxis  RotationAngleUnits=rad  RotationStandardAxis=+Z  RotationAngle=pi/2  RotationArbitraryAxis=[0, 0, 1]  FollAlignAxisA=+X  BaseAlignAxisA=+Y  FollAlignAxisB=+Y  BaseAlignAxisB=+Z  RotationSequenceAxes=FollowerAxes  RotationSequence=XYX  RotationSequenceAngles=[0 0 0]  RotationSequenceAnglesUnits=deg  RotationMatrix=[1 0 0; 0 1 0; 0 0 1]
  Wx : PMIOPort  Side=Left
  Wy : PMIOPort  Port=2  Side=Right
  connections:
  jRightShoulder_rotx_AxisInvTransform3/RConn1 -- Wy/RConn1
  jRightShoulder_rotx_AxisInvTransform2/RConn1 -- jRightShoulder_rotx_AxisInvTransform3/LConn1
  Wx/RConn1 -- jRightShoulder_rotx_AxisInvTransform2/LConn1

== system master_thesis_simulink/System/Human arm/Wrist_joint/Wy_Wz ==
  jRightShoulder_roty_AxisInvTransform : sm_lib/Frames and Transforms/Rigid Transform  TranslationMethod=Cartesian  TranslationStandardOffset=0  TranslationLengthUnit=m  TranslationStandardAxis=+Z  TranslationCartesianOffset=[0, 0, 0]  TranslationROffset=0  TranslationROffsetUnits=m  TranslationZOffset=0  TranslationZOffsetUnits=m  TranslationThetaOffset=0  TranslationThetaOffsetUnits=deg  RotationMethod=ArbitraryAxis  RotationAngleUnits=rad  RotationStandardAxis=+Z  RotationAngle=pi/2  RotationArbitraryAxis=[0, 1, 0]  FollAlignAxisA=+X  BaseAlignAxisA=+Y  FollAlignAxisB=+Y  BaseAlignAxisB=+Z  RotationSequenceAxes=FollowerAxes  RotationSequence=XYX  RotationSequenceAngles=[0 0 0]  RotationSequenceAnglesUnits=deg  RotationMatrix=[1 0 0; 0 1 0; 0 0 1]
  jRightShoulder_roty_AxisInvTransform1 : sm_lib/Frames and Transforms/Rigid Transform  TranslationMethod=Cartesian  TranslationStandardOffset=0  TranslationLengthUnit=m  TranslationStandardAxis=+Z  TranslationCartesianOffset=[0, 0, 0]  TranslationROffset=0  TranslationROffsetUnits=m  TranslationZOffset=0  TranslationZOffsetUnits=m  TranslationThetaOffset=0  TranslationThetaOffsetUnits=deg  RotationMethod=ArbitraryAxis  RotationAngleUnits=rad  RotationStandardAxis=+Z  RotationAngle=pi/2  RotationArbitraryAxis=[0, 0, 1]  FollAlignAxisA=+X  BaseAlignAxisA=+Y  FollAlignAxisB=+Y  BaseAlignAxisB=+Z  RotationSequenceAxes=FollowerAxes  RotationSequence=XYX  RotationSequenceAngles=[0 0 0]  RotationSequenceAnglesUnits=deg  RotationMatrix=[1 0 0; 0 1 0; 0 0 1]
  Wy : PMIOPort  Side=Left
  Wz : PMIOPort  Port=2  Side=Right
  connections:
  Wz/RConn1 -- jRightShoulder_roty_AxisInvTransform1/RConn1
  Wy/RConn1 -- jRightShoulder_roty_AxisInvTransform/LConn1
  jRightShoulder_roty_AxisInvTransform/RConn1 -- jRightShoulder_roty_AxisInvTransform1/LConn1

== system master_thesis_simulink/System/Show Results/EKF/Human arm ==
  note: B_shoulder
  note: SHOULDER
  note: ELBOW-FOREARM
  note: WRIST-HAND
  q_EKF : Inport
  Demux : Demux  Outputs=7
  Elbow_joint : Subsystem
  Markers : Subsystem  Commented=on
  Mechanism Configuration : sm_lib/Utilities/Mechanism Configuration  UniformGravity=Constant  GravityVector=[0 0 -9.80665]  GravityUnits=m/s^2  LinearizationDelta=0.001  JointModeTransitionNonlinearIterations=2
  Mux2 : Mux  Inputs=3
  Mux3 : Mux  Inputs=3
  RightForeArm : Subsystem
  RightHand : Subsystem
  RightShoulder : Subsystem
  RightShoulder_joint : Subsystem
  Solver Configuration1 : nesl_utility/Solver Configuration  PhysicalDomain=network_engine_domain  SubClassName=solver  LeftPortType=input  RightPortType=generic  Tones=[]  Harmonics=[]  SimulateNoise=off  Profile=off  UseLocalSampling=off  EnableSwitchedLinearOptims=on  FrequencyDomain=off  UseCCode=off  RelTol=0.001  AbsTol=0.001  MinStep=1e-09  ToWorkspace=off  RevertToSquareIcSolve=off  NumHomotopyIterations=100  PhasorMode=off  PhasorModeNumHarmonics=1  IndexReductionMethod=DerivativeReplacement  DoDC=off  ResidualTolerance=1e-09  UseLocalSolver=off  LocalSolverChoice=NE_BACKWARD_EULER_ADVANCER  LocalSolverSampleTime=0.001  DoFixedCost=off  MaxNonlinIter=3  MaxModeIter=2  ComputeImpulses=off  ImpulseIterations=2  LinearAlgebra=auto  LinearAlgebraNumThread=0  EquationFormulation=NE_TIME_EF  DelaysMemoryBudget=1024  AutomaticFiltering=on  FilteringTimeConstant=0.001  PartitionStorageMethod=AS_NEEDED  PartitionMemoryBudget=1024  PartitionMethod=ROBUST
      settings: SourceProductBaseCode=SS,PW,VE
  World Frame : sm_lib/Frames and Transforms/World Frame
  Wrist_joint : Subsystem
  wires:
  q_EKF/1 -> Demux/1
  Demux/1 -> Mux2/1
  Demux/2 -> Mux2/2
  Demux/3 -> Mux2/3
  Mux2/1 -> [q_sh]
  Demux/4 -> [q_fo]
  Mux3/1 -> [q_ha]
  Demux/7 -> Mux3/3
  Demux/6 -> Mux3/2
  Demux/5 -> Mux3/1
  [q_sh] -> RightShoulder_joint/1(Input)
  [q_fo] -> Elbow_joint/1(Input)
  [q_ha] -> Wrist_joint/1(Input)
  connections:
  RightShoulder/LConn1 -- RightShoulder_joint/RConn1
  RightHand/LConn1 -- Wrist_joint/RConn1
  Elbow_joint/LConn1 -- RightShoulder/RConn1
  Wrist_joint/LConn1 -- RightForeArm/RConn1
  RightForeArm/LConn2 -- RightHand/LConn2 -- RightShoulder/LConn2 -- World Frame/RConn1 -- Mechanism Configuration/RConn1 -- RightShoulder_joint/LConn1 -- Solver Configuration1/RConn1
  Elbow_joint/RConn1 -- RightForeArm/LConn1
